simulink model "NandiniG_23EEM1S02_foc_3mli_working_fine_Moscap"  (R2024b)
settings: Solver=ode1  StartTime=0.0  StopTime=1  FixedStep=0.000001  MaxStep=1e-4  RelTol=1e-3
InitFcn:
  | fs=2000;
model workspace (MAT data in the model file):
  Vref = 440
  cutoff_frequency = 500
  damping_factor = 0.707
  fn = 100
  fs = 2000
  ma = 1
libraries: simulink x24, spsMosfetLib x12, spsVoltageMeasurementLib x10, spsDiodeLib x6, powerlib_extras x6, spsSeriesRLCBranchLib x4, spsCurrentMeasurementLib x3, slpidlib x3, spsIGBTDiodeLib x2, spsDCVoltageSourceLib x1, spsGroundLib x1, spsPermanentMagnetSynchronousMachineLib x1
(part 2 of 2)

== matlab function NandiniG_23EEM1S02_foc_3mli_working_fine_Moscap/3- Level NPC/NPC 3-level inverter/Subsystem2/MATLAB Function ==
  settings: updateMethod=DISCRETE
  data: inputSignal input; peak output; currentTime input
function peak = getPeak(inputSignal, currentTime)
    % GETPEAK Function to track the peak value of a running waveform.
    %
    % INPUT:
    % inputSignal - Current sample of the waveform.
    % currentTime - Current simulation time.
    %
    % OUTPUT:
    % peak - The maximum absolute value encountered so far.
 
    % Persistent variables to store the peak values and the reset flag
    persistent maxPeak minPeak resetDone;
 
    % Initialize the persistent variables on the first function call
    if isempty(maxPeak)
        maxPeak = -inf;  % Start with a very low value
    end
    if isempty(minPeak)
        minPeak = inf;   % Start with a very high value
    end
    if isempty(resetDone)
        resetDone = false;  % Flag to indicate if reset has been done
    end
 
    % Reset the peak values once at 0.1 seconds
    if currentTime >= 0.11 && ~resetDone
        maxPeak = -inf;
        minPeak = inf;
        resetDone = true;  % Set the flag to true after reset
    end
 
    % Update the peak values if the current sample is larger or smaller
    if inputSignal > maxPeak
        maxPeak = inputSignal;
    end
    if inputSignal < minPeak
        minPeak = inputSignal;
    end
 
    % Calculate the peak-to-peak value
    peak = max(abs(maxPeak), abs(minPeak));
end
